simulink model "sim_21uec072"  (R2022b)
settings: Solver=VariableStepAuto  StartTime=0.0  StopTime=0  RelTol=1e-3
values from neighbouring files (symbols this model uses):
  N_sd = 1/sqrt(snr_lin)    [task1.m]    (also in task4.m = 0.01; task5.m = 0.01; task6.m = 1./sqrt(snr_lin))
settings Model: Creator=DSP-35  LastModifiedBy=DSP-35

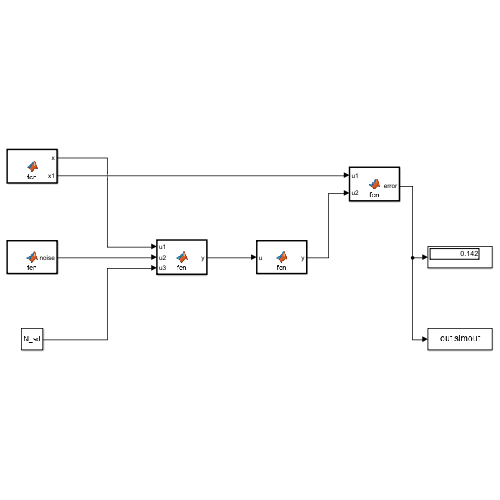
[thumbnail: Simulink's stored preview of the top-level diagram]
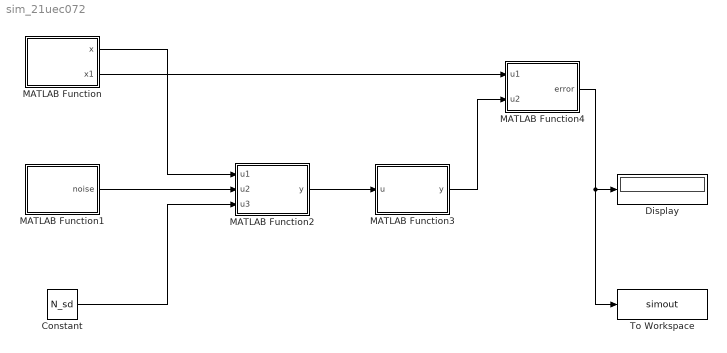
== system sim_21uec072 ==
  Constant : Constant  Value=N_sd
  Display : Display
  MATLAB Function : MATLAB Function  TreatAsAtomicUnit=on
  MATLAB Function1 : MATLAB Function  TreatAsAtomicUnit=on
  MATLAB Function2 : MATLAB Function  TreatAsAtomicUnit=on
  MATLAB Function3 : MATLAB Function  TreatAsAtomicUnit=on
  MATLAB Function4 : MATLAB Function  TreatAsAtomicUnit=on
  To Workspace : ToWorkspace  VariableName=simout  SampleTime=-1
      settings: Save2DSignal=2-D array (concatenate along first dimension)
  wires:
  MATLAB Function/1(x) -> MATLAB Function2/1(u1)
  MATLAB Function1/1(noise) -> MATLAB Function2/2(u2)
  Constant/1 -> MATLAB Function2/3(u3)
  MATLAB Function4/1(error) -> To Workspace/1, Display/1
  MATLAB Function2/1(y) -> MATLAB Function3/1(u)
  MATLAB Function3/1(y) -> MATLAB Function4/2(u2)
  MATLAB Function/2(x1) -> MATLAB Function4/1(u1)

== matlab function sim_21uec072/MATLAB Function ==
  data: x output; x1 output
function [x,x1] = fcn()

N = 1e3;
x1 = randi(2,1,N) - 1;
x = 2*(x1) - 1;

== matlab function sim_21uec072/MATLAB Function2 ==
  data: u1 input; y output; u2 input; u3 input
function y = fcn(u1,u2,u3)

N = 1e3;
y = u1 + u2*u3;

== matlab function sim_21uec072/MATLAB Function3 ==
  data: u input; y output
function y = fcn(u)

y = u>0;

== matlab function sim_21uec072/MATLAB Function4 ==
  data: u1 input; error output; u2 input
function error = fcn(u1, u2)

N = 1e3;
error = sum(abs(u1 - u2).^2)/N;

== matlab function sim_21uec072/MATLAB Function1 ==
  data: noise output
function noise = fcn()

N = 1e3;
noise = complex(randn(1,N),randn(1,N));
